simulink model "modelo_motor"  (R2022b)
settings: Solver=VariableStepAuto  StartTime=0.0  StopTime=10.0  RelTol=1e-3
values from neighbouring files (symbols this model uses):
  airgap_drag = [8 13 18 23]    [datos_modelo.mat]
  Force_drag = [-0.0263599613947 43.4567385798 79.8814932025 112.890713456 143.193346103 171.145741633 196.959308063 220.848934943 -0.0285293042528 24.6775545387 45.2474492116 63.9699604043 ... (32 elements, 8x4)]    [datos_modelo.mat]
  frecuencia = (3:3:48)    [carga_datos_motor_simple.m]    (also in datos_modelo.mat = [3 6 9 12 15 18 21 24 27 30 33 36 ... (16 elements, 1x16)])
  frecuencia_freno = -48:3:-3    [carga_datos_frenado_v3.m]    (also in carga_datos_frenado_v4.m; datos_modelo.mat = [-48 -45 -42 -39 -36 -33 -30 -27 -24 -21 -18 -15 ... (16 ele)
  FuerzaX_acel = []    [carga_datos_motor_simple.m]    (also in datos_modelo.mat = [0.156686825585 1.1015935563 2.01038201102 2.86930542934 3.6)
  FuerzaX_freno = []    [carga_datos_frenado_v3.m]    (also in datos_modelo.mat = [153.020892613 -180.239809195 -245.613894698 -262.756397176 )
  FuerzaY_acel = []    [carga_datos_motor_simple.m]    (also in datos_modelo.mat = [16.7719587108 16.6669307493 16.4360183454 16.0997979621 15.)
  Ipeak = (10:10:100)    [carga_datos_fuerza_laterales.m]    (also in carga_datos_motor_simple.m; datos_modelo.mat = [10 20 30 40 50 60 70 80 90 100])
  L = [0.00288301128086 0.00287460594326 0.00286413458194 0.00286292567045 0.00283652697085 0.00271657977235 0.0024764202896 0.0021234760901 0.00287319201871 0.00287259972172 0.0028679034407 0.0028580918991 ... (1408 elements, 8x11x16)]    [datos_modelo.mat]
  mass = 200    [datos_modelo.mat]
  pole_length = 0.114    [datos_modelo.mat]
  r = 0.384    [datos_modelo.mat]
  slip = (1:-0.1:0)    [carga_datos_motor_simple.m]    (also in datos_modelo.mat = [0 0.1 0.2 0.3 0.4 0.5 0.6 0.7 0.8 0.9 1])
  slip_freno = 1.1:0.1:2    [carga_datos_frenado_v4.m]
  vel_drag = [0 5 10 15 20 25 30 35]    [datos_modelo.mat]
settings Model: Creator=mique  LastModifiedBy=mique

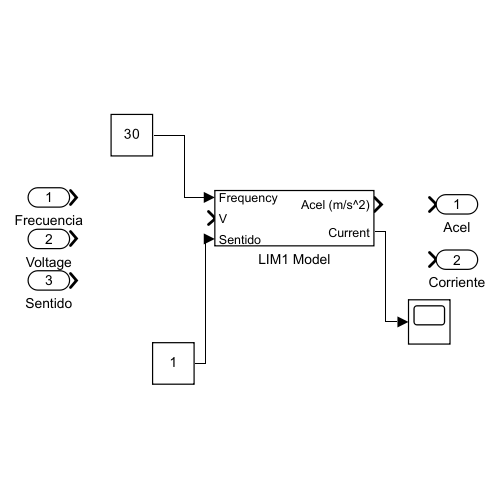
[thumbnail: Simulink's stored preview of the top-level diagram]
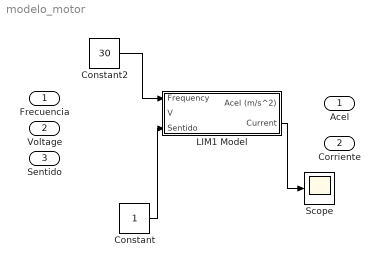
== system modelo_motor ==
  Frecuencia : Inport
  Voltage : Inport  Port=2
  Sentido : Inport  Port=3
  Constant : Constant
  Constant2 : Constant  Value=30
  LIM1 Model : Subsystem
  Scope : Scope
  Acel : Outport
  Corriente : Outport  Port=2
  wires:
  Constant/1 -> LIM1 Model/3(Sentido)
  Constant2/1 -> LIM1 Model/1(Frequency)
  LIM1 Model/2(Current) -> Scope/1

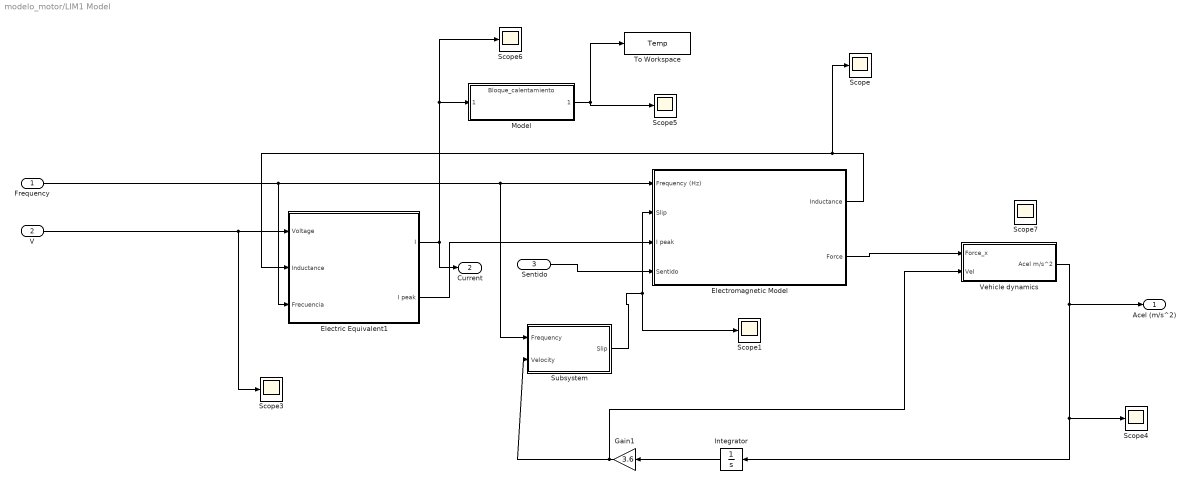
== system modelo_motor/LIM1 Model ==
  Frequency : Inport
  "V " : Inport  Port=2
  Sentido : Inport  Port=3
  Electric Equivalent1 : Subsystem
  Electromagnetic Model : Subsystem
  Gain1 : Gain  Gain=3.6
  Integrator : Integrator
  Model : ModelReference  ModelNameDialog=Bloque_calentamiento.slx  SimulationMode=Normal  ModelReferenceVersion=3.8
  Scope{,1,3..7} (7 alike) : Scope
  Subsystem : Subsystem
  To Workspace : ToWorkspace  VariableName=Temp  SampleTime=-1
  Vehicle dynamics : Subsystem
  Acel (m/s^2) : Outport
  Current : Outport  Port=2
  wires:
  Vehicle dynamics/1(Acel m/s^2) -> Integrator/1, Scope4/1, Acel (m/s^2)/1
  Electric Equivalent1/2(I peak) -> Electromagnetic Model/3(I peak)
  Electromagnetic Model/1(Inductance) -> Scope/1, Electric Equivalent1/2(Inductance)
  Frequency/1 -> Electric Equivalent1/3(Frecuencia), Subsystem/1(Frequency), Electromagnetic Model/1(Frequency (Hz))
  Integrator/1 -> Gain1/1
  "V "/1 -> Scope3/1, Electric Equivalent1/1(Voltage)
  Model/1 -> Scope5/1, To Workspace/1
  Electric Equivalent1/1("I ") -> Current/1, Scope6/1, Model/1
  Sentido/1 -> Electromagnetic Model/4(Sentido)
  Subsystem/1(Slip) -> Scope1/1, Electromagnetic Model/2(Slip)
  Gain1/1 -> Vehicle dynamics/2(Vel), Subsystem/2(Velocity)
  Electromagnetic Model/2(Force) -> Vehicle dynamics/1(Force_x)

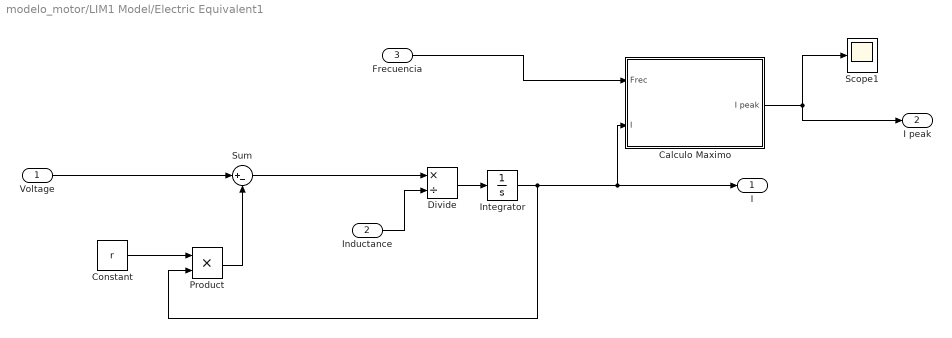
== system modelo_motor/LIM1 Model/Electric Equivalent1 ==
  Voltage : Inport
  Inductance : Inport  Port=2
  Frecuencia : Inport  Port=3
  Calculo Maximo : Subsystem
  Constant : Constant  Value=r
  Divide : Product  Inputs=*/
  Integrator : Integrator
  Product : Product
  Scope1 : Scope
  Sum : Sum  Inputs=|+-
  "I " : Outport
  I peak : Outport  Port=2
  wires:
  Voltage/1 -> Sum/1
  Integrator/1 -> Calculo Maximo/2(I), "I "/1, Product/2
  Constant/1 -> Product/1
  Product/1 -> Sum/2
  Divide/1 -> Integrator/1
  Sum/1 -> Divide/1
  Inductance/1 -> Divide/2
  Calculo Maximo/1(I peak) -> I peak/1, Scope1/1
  Frecuencia/1 -> Calculo Maximo/1(Frec)

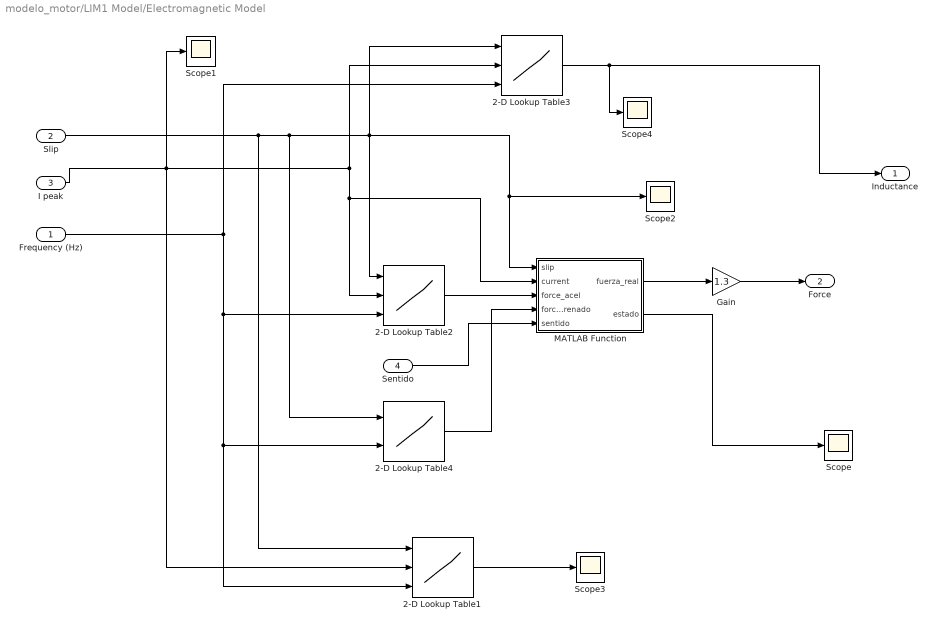
== system modelo_motor/LIM1 Model/Electromagnetic Model ==
  Frequency (Hz) : Inport
  Slip : Inport  Port=2
  I peak : Inport  Port=3
  Sentido : Inport  Port=4
  2-D Lookup Table1 : Lookup_n-D  NumberOfTableDimensions=3  BreakpointsForDimension1=slip  BreakpointsForDimension2=Ipeak  BreakpointsForDimension3=frecuencia  Table=FuerzaY_acel  InterpMethod=Nearest  InternalRulePriority=Speed  RndMeth=Simplest
      settings: InputPortMap=u0,u1,u2
  2-D Lookup Table2 : Lookup_n-D  NumberOfTableDimensions=3  BreakpointsForDimension1=slip  BreakpointsForDimension2=Ipeak  BreakpointsForDimension3=frecuencia  Table=FuerzaX_acel  InterpMethod=Nearest  InternalRulePriority=Speed  RndMeth=Simplest
      settings: InputPortMap=u0,u1,u2
  2-D Lookup Table3 : Lookup_n-D  NumberOfTableDimensions=3  BreakpointsForDimension1=Ipeak(2:(end-1))  BreakpointsForDimension2=slip  BreakpointsForDimension3=frecuencia  Table=L  InterpMethod=Nearest  InternalRulePriority=Speed  RndMeth=Simplest
      settings: InputPortMap=u0,u1,u2
  2-D Lookup Table4 : Lookup_n-D  BreakpointsForDimension1=slip_freno  BreakpointsForDimension2=frecuencia_freno  BreakpointsForDimension3=frecuencia  Table=FuerzaX_freno  InterpMethod=Nearest  InternalRulePriority=Speed  RndMeth=Simplest
      settings: InputPortMap=u0,u1
  Gain : Gain  Gain=1.3
  MATLAB Function : MATLAB Function  TreatAsAtomicUnit=on
  Scope{,1..4} (5 alike) : Scope
  Inductance : Outport
  Force : Outport  Port=2
  wires:
  2-D Lookup Table3/1 -> Scope4/1, Inductance/1
  Frequency (Hz)/1 -> 2-D Lookup Table4/2, 2-D Lookup Table1/3, 2-D Lookup Table2/3, 2-D Lookup Table3/3
  I peak/1 -> 2-D Lookup Table1/2, MATLAB Function/2(current), 2-D Lookup Table2/2, 2-D Lookup Table3/2, Scope1/1
  Slip/1 -> 2-D Lookup Table1/1, 2-D Lookup Table4/1, Scope2/1, MATLAB Function/1(slip), 2-D Lookup Table2/1, 2-D Lookup Table3/1
  2-D Lookup Table2/1 -> MATLAB Function/3(force_acel)
  2-D Lookup Table1/1 -> Scope3/1
  2-D Lookup Table4/1 -> MATLAB Function/4(force_frenado)
  Sentido/1 -> MATLAB Function/5(sentido)
  MATLAB Function/2(estado) -> Scope/1
  MATLAB Function/1(fuerza_real) -> Gain/1
  Gain/1 -> Force/1

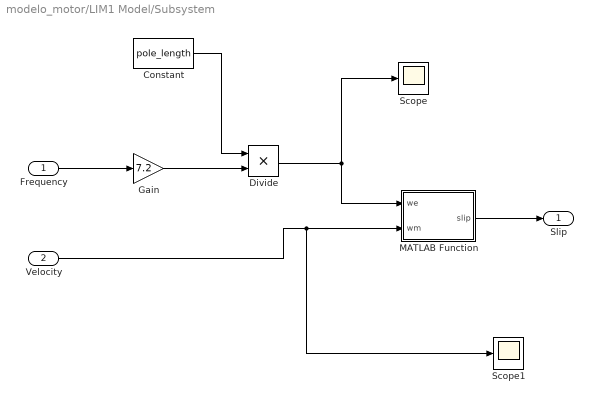
== system modelo_motor/LIM1 Model/Subsystem ==
  Frequency : Inport
  Velocity : Inport  Port=2
  Constant : Constant  Value=pole_length
  Divide : Product  Inputs=**
  Gain : Gain  Gain=7.2
  MATLAB Function : MATLAB Function  TreatAsAtomicUnit=on
  Scope : Scope
  Scope1 : Scope
  Slip : Outport
  wires:
  Frequency/1 -> Gain/1
  MATLAB Function/1(slip) -> Slip/1
  Gain/1 -> Divide/2
  Constant/1 -> Divide/1
  Divide/1 -> Scope/1, MATLAB Function/1(we)
  Velocity/1 -> Scope1/1, MATLAB Function/2(wm)

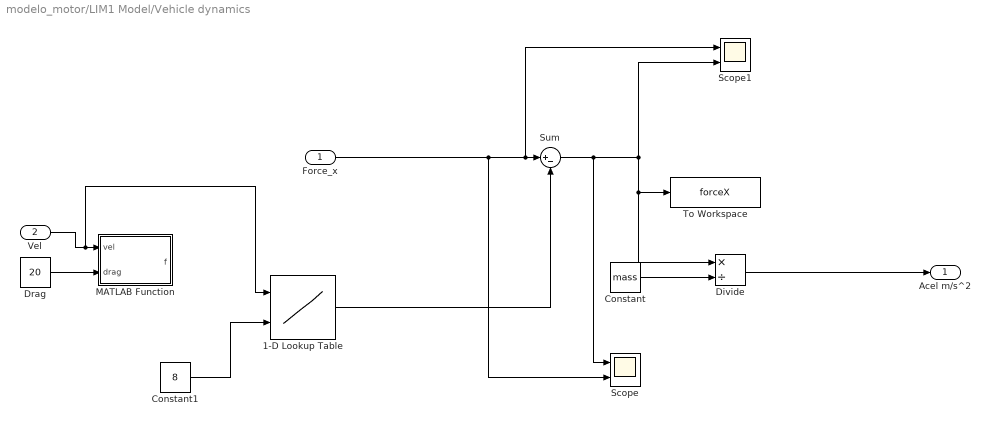
== system modelo_motor/LIM1 Model/Vehicle dynamics ==
  Force_x : Inport
  Vel : Inport  Port=2
  1-D Lookup Table : Lookup_n-D  BreakpointsForDimension1=vel_drag  BreakpointsForDimension2=airgap_drag  Table=Force_drag  InterpMethod=Nearest  InternalRulePriority=Speed  RndMeth=Simplest
      settings: InputPortMap=u0,u1
  Constant : Constant  Value=mass
  Constant1 : Constant  Value=8
  Divide : Product  Inputs=*/
  Drag : Constant  Value=20
  MATLAB Function : MATLAB Function  TreatAsAtomicUnit=on
  Scope : Scope  NumInputPorts=2
  Scope1 : Scope  NumInputPorts=2
  Sum : Sum  Inputs=|+-
  To Workspace : ToWorkspace  VariableName=forceX  SampleTime=-1
  Acel m/s^2 : Outport
  wires:
  Divide/1 -> Acel m/s^2/1
  Constant/1 -> Divide/2
  Force_x/1 -> Scope/2, Scope1/1, Sum/1
  Sum/1 -> Scope/1, Scope1/2, Divide/1, To Workspace/1
  Drag/1 -> MATLAB Function/2(drag)
  Vel/1 -> 1-D Lookup Table/1, MATLAB Function/1(vel)
  1-D Lookup Table/1 -> Sum/2
  Constant1/1 -> 1-D Lookup Table/2

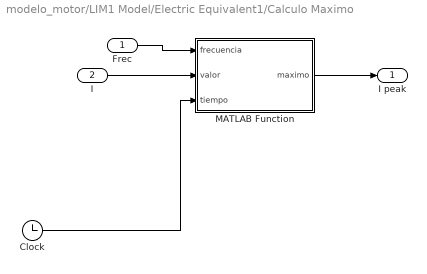
== system modelo_motor/LIM1 Model/Electric Equivalent1/Calculo Maximo ==
  Frec : Inport
  I : Inport  Port=2
  Clock : Clock
  MATLAB Function : MATLAB Function  TreatAsAtomicUnit=on
  I peak : Outport
  wires:
  Frec/1 -> MATLAB Function/1(frecuencia)
  I/1 -> MATLAB Function/2(valor)
  MATLAB Function/1(maximo) -> I peak/1
  Clock/1 -> MATLAB Function/3(tiempo)

== matlab function modelo_motor/LIM1 Model/Electromagnetic Model/MATLAB Function ==
  data: slip input; fuerza_real output; current input; force_acel input; force_frenado input; sentido input; estado output
function [fuerza_real,estado]= fcn(slip,current,force_acel,force_frenado,sentido)

if sentido>=0
    force=force_acel;
    estado=1;
else
    force=force_frenado;
    estado=2;
end

if slip == 0 || current<2 && current>-2

    fuerza_real=0;
    estado=3;

else
    fuerza_real=force;
    estado=4;
end

== matlab function modelo_motor/LIM1 Model/Electric Equivalent1/Calculo Maximo/MATLAB Function ==
  settings: updateMethod=DISCRETE
  data: frecuencia input; maximo output; valor input; tiempo input
function maximo = fcn(frecuencia,valor,tiempo)

   persistent antiguo_maximo
    if isempty(antiguo_maximo)
       antiguo_maximo=0;
    end
    persistent t_maximo
    if isempty(t_maximo)
       t_maximo=0;
    end

periodo=1/abs(frecuencia);


if abs(valor)>=antiguo_maximo
    maximo=abs(valor);
    antiguo_maximo=abs(valor);
    t_maximo=tiempo;
else
    maximo=antiguo_maximo;
    if tiempo>t_maximo+periodo
        maximo=abs(valor);
        antiguo_maximo=abs(valor);
        t_maximo=tiempo;
    end
end

== matlab function modelo_motor/LIM1 Model/Subsystem/MATLAB Function ==
  data: we input; slip output; wm input
function slip = fcn(we,wm)

slip = (we-wm)/we;

== matlab function modelo_motor/LIM1 Model/Vehicle dynamics/MATLAB Function ==
  data: vel input; f output; drag input
function f = fcn(vel,drag)

if vel > 5
    f=drag;
else
    f=0;
end
